simulink model "Sim42"  (R2019a)
settings: Solver=FixedStepAuto  StartTime=0.0  StopTime=10.0  FixedStep=0.0001  RelTol=1e-3
undefined symbols (not defined in the file): magnitude
settings Model: Creator=fbleo  LastModifiedBy=fbleo

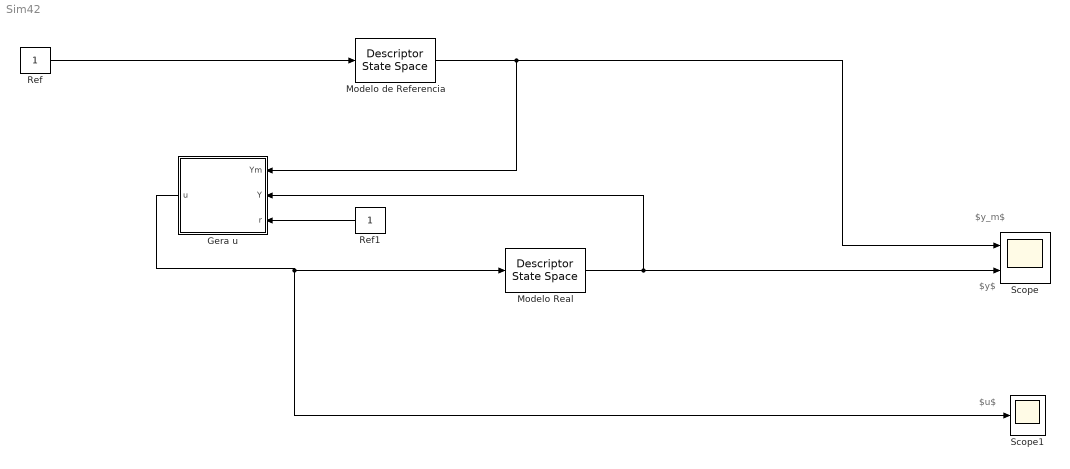
== system Sim42 ==
  note: $y_m$
  note: $y$
  note: $u$
  Gera u : Subsystem
  Modelo Real : DescriptorStateSpace  A=-1  B=2  D=0  InitialCondition=0.5
  Modelo de Referencia : DescriptorStateSpace  A=-3  B=3  D=0  InitialCondition=0
  Ref : Constant
  Ref1 : Constant
  Scope : Scope  NumInputPorts=2
  Scope1 : Scope
  wires:
  Modelo de Referencia/1 -> Scope/1, Gera u/1(Ym)
  Gera u/1(u) -> Modelo Real/1, Scope1/1
  Modelo Real/1 -> Gera u/2(Y), Scope/2
  Ref/1 -> Modelo de Referencia/1
  Ref1/1 -> Gera u/3(r)

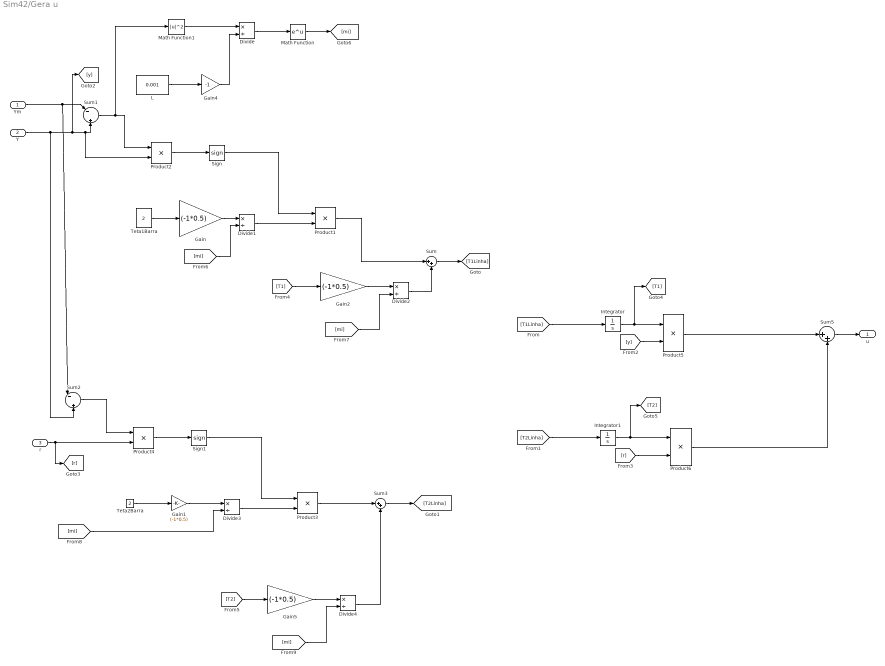
== system Sim42/Gera u ==
  Ym : Inport
  Y : Inport  Port=2
  r : Inport  Port=3
  Divide{,1..4} (5 alike) : Product  Inputs=*/
  Gain{,1..2,5} (4 alike) : Gain  Gain=(-1*0.5)
  Gain4 : Gain  Gain=-1
  Integrator : Integrator  InitialCondition=-0.65
  Integrator1 : Integrator  InitialCondition=1.14
  L : Constant  Value=0.001
  Math Function : Math  SaturateOnIntegerOverflow=on
  Math Function1 : Math  Operator=magnitude^2  SaturateOnIntegerOverflow=on
  Product{1..6} (6 alike) : Product
  Sign : Signum
  Sign1 : Signum
  Sum : Sum  Inputs=|++
  Sum1 : Sum  Inputs=|-||+
  Sum2 : Sum  Inputs=|-||+
  Sum3 : Sum  Inputs=|++
  Sum5 : Sum  Inputs=|++
  Teta1Barra : Constant  Value=2
  Teta2Barra : Constant  Value=2
  u : Outport
  wires:
  Sign/1 -> Product1/1
  Teta1Barra/1 -> Gain/1
  Sum1/1 -> Math Function1/1, Product2/1
  Product2/1 -> Sign/1
  Product1/1 -> Sum/1
  Ym/1 -> Sum1/1, Sum2/1
  Sign1/1 -> Product3/1
  Product4/1 -> Sign1/1
  Sum2/1 -> Product4/1
  Y/1 -> [y], Product2/2, Sum1/2, Sum2/2
  Teta2Barra/1 -> Gain1/1
  r/1 -> [r], Product4/2
  [y] -> Product5/2
  [T1Linha] -> Integrator/1
  [T2Linha] -> Integrator1/1
  [r] -> Product6/2
  Product5/1 -> Sum5/1
  Product6/1 -> Sum5/2
  Sum5/1 -> u/1
  Sum/1 -> [T1Linha]
  Integrator/1 -> [T1], Product5/1
  [T1] -> Gain2/1
  Integrator1/1 -> [T2], Product6/1
  Product3/1 -> Sum3/1
  Sum3/1 -> [T2Linha]
  L/1 -> Gain4/1
  Math Function1/1 -> Divide/1
  Gain4/1 -> Divide/2
  Divide/1 -> Math Function/1
  Math Function/1 -> [mi]
  Gain/1 -> Divide1/1
  [mi] -> Divide1/2
  [mi] -> Divide2/2
  Gain2/1 -> Divide2/1
  Divide2/1 -> Sum/2
  Divide1/1 -> Product1/2
  Divide3/1 -> Product3/2
  [mi] -> Divide3/2
  Gain1/1 -> Divide3/1
  [T2] -> Gain5/1
  Divide4/1 -> Sum3/2
  Gain5/1 -> Divide4/1
  [mi] -> Divide4/2
